simulink model "hw2p2a"  (R2017a)
settings: Solver=FixedStepAuto  StartTime=0.0  StopTime=10.0  FixedStep=0.1  RelTol=1e-3
settings Model: Creator=Soutrik  LastModifiedBy=Soutrik

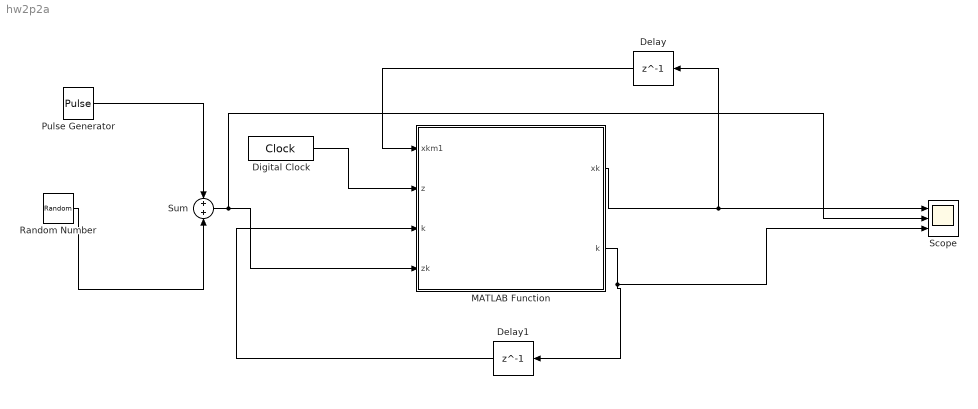
== system hw2p2a ==
  Delay : Delay  DelayLength=1  InitialCondition=0  SampleTime=0.1
  Delay1 : Delay  DelayLength=1  InitialCondition=0  SampleTime=0.1
  Digital Clock : DigitalClock  SampleTime=0.1
  MATLAB Function : MATLAB Function  TreatAsAtomicUnit=on
  Pulse Generator : DiscretePulseGenerator  PulseType=Time based  Period=5  PulseWidth=50
  Random Number : RandomNumber  Variance=0.005  SampleTime=0.1
  Scope : Scope  NumInputPorts=3
  Sum : Sum
  wires:
  Pulse Generator/1 -> Sum/1
  Random Number/1 -> Sum/2
  MATLAB Function/1(xk) -> Delay/1, Scope/1
  Sum/1 -> Scope/2, MATLAB Function/4(zk)
  Delay/1 -> MATLAB Function/1(xkm1)
  MATLAB Function/2(k) -> Scope/3, Delay1/1
  Digital Clock/1 -> MATLAB Function/2(z)
  Delay1/1 -> MATLAB Function/3("k ")

== matlab function hw2p2a/MATLAB Function ==
  data: xkm1 input; z input; k input; xk output; zk input; k output
function [xk,k]= fcn(xkm1,z,k,zk)

  if z< 0.2
      k=1;
  else
      k=k+1;
  end
  
  if k>9
      k=9;
  end

  xk=xkm1+(1/k)*(zk-xkm1);
